simulink model "NuevosModelos"  (R2024b)
settings: Solver=VariableStepAuto  StartTime=0.0  StopTime=10.0  RelTol=1e-3
values from neighbouring files (symbols this model uses):
  K_motor = 0.001514    [ParametrosParaSimulink.m]
  tau_motor = 0.593    [ParametrosParaSimulink.m]
settings Model: Creator=lucas  LastModifiedBy=lucas

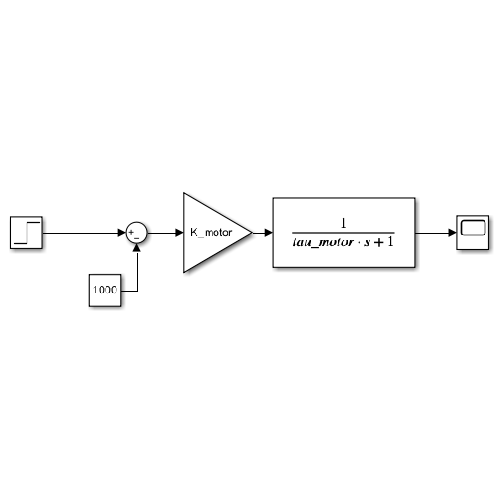
[thumbnail: Simulink's stored preview of the top-level diagram]
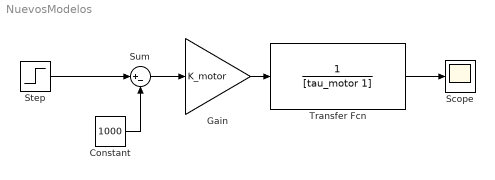
== system NuevosModelos ==
  Constant : Constant  Value=1000
  Gain : Gain  Gain=K_motor
  Scope : Scope
  Step : Step  Time=0  After=1500  SampleTime=0
  Sum : Sum  Inputs=|+-
  Transfer Fcn : TransferFcn  Denominator=[tau_motor 1]
  wires:
  Gain/1 -> Transfer Fcn/1
  Transfer Fcn/1 -> Scope/1
  Step/1 -> Sum/1
  Sum/1 -> Gain/1
  Constant/1 -> Sum/2
